simulink model "AGTF30SysDyn_PExPIn"  (R2023b)
settings: Solver=ode4  StartTime=0.0  StopTime=MWS.In.tend  FixedStep=MWS.In.Ts  RelTol=1e-3  EnableMultiTasking=on
model workspace: external: MAT-File (data not in the file)
values from neighbouring files (symbols this model uses):
  MWS = setup_initialize(MWS,startPt,SSsolverSP)    [Setup_Simulation.m]    (also in run_AGTF30e_script.m = Setup_Simulation(inputMethod,MWS.In,filename,Mdl,SSsolverSP))
undefined symbols (not defined in the file or in its folder): DiscIntNeverNeededParam
libraries: simulink x32, Lib_Solve_ModelSource_TMATS x28, Lib_EMTAT x27, Lib_Cntrl_FirstOrderSensor_TMATS x19, Lib_Cntrl_FirstOrderActuator_TMATS x2, Lib_Cntrl_LimitSelect_TMATS x2, Lib_Solve_OuterLoopIntegrator_TMATS x2, Lib_Cntrl_CorrectedSpeed_TMATS x1, Lib_Solve_IterNRSolverJC_TMATS x1, slpidlib x1
(part 7 of 8)

== system AGTF30SysDyn_PExPIn/Control System/Electric Machine Controllers/EM Controllers/PGB EM Control/VEATE EM Controllers/Base Power/Base Power - Boost and PEx/Boost PEx - HC LR CS ==
  note: COUPLING EM
  note: HP - CARRIER , LP - RING, COUPLING - SUN
  note: LP EM
  note: HP EM
  note: MAKE SURE THE POWER DEMAND/LOAD IS BEING
      | PROVIDED. WITH VEATE, CROSS-COUPLING EFFECTS
      | IN THE COMPONENTS CAN RELECT POWER BACK TO
      | OTHER COMPONENTS AND A SMALL DIFFERENCE (A FEW
      | 10'S OF HORSEPOWER) COULDBE OBSERVED. THIS WILL
      | WIPE OUT THE DIFFENCE.
  PwrL_Base : Inport
  PwrH_Base : Inport  Port=2
  K_PXeffL : Inport  Port=3
  K_PXeffH : Inport  Port=4
  NS : Inport  Port=5
  NR : Inport  Port=6
  NC : Inport  Port=7
  Abs : Abs  SaturateOnIntegerOverflow=off
  Abs1 : Abs  SaturateOnIntegerOverflow=off
  Abs2 : Abs  SaturateOnIntegerOverflow=off
  Divide : Product  Inputs=*/
  Divide{2..3,5..7,9..11} (8 alike) : Product  Inputs=**
  Gain1 : Gain  Gain=1/5252.113
  Gain15 : Gain  Gain=1/MWS.Shaft.PGB.Ring.GR_gb %GR_gb = Ngb/Nem
  Gain2 : Gain  Gain=1/5252.113
  Gain3 : Gain  Gain=1/MWS.Shaft.PGB.Carrier.GR_gb %GR_gb = Ngb/Nem
  Gain4 : Gain  Gain=1/5252.113
  Gain5 : Gain  Gain=1/MWS.Shaft.PGB.Sun.GR_gb %GR_gb = Ngb/Nem
  MinMax : MinMax
  MinMax1 : MinMax
  MinMax2 : MinMax
  Mux1 : Mux  Inputs=3
  Mux2 : Mux  Inputs=3
  Mux3 : Mux  Inputs=3
  PwrMax_Base : Constant  Value=MWS.Cntrl.EMR.PwrMax_Base
  PwrMax_Base1 : Constant  Value=MWS.Cntrl.EMC.PwrMax_Base
  PwrMax_Base2 : Constant  Value=MWS.Cntrl.EMS.PwrMax_Base
  Sign : Signum
  Sign1 : Signum
  Sign2 : Signum
  Sum : Sum  Inputs=|+-
  Sum1 : Sum  Inputs=|-+
  Sum5 : Sum  Inputs=|+++
  Sum6 : Sum  Inputs=|++
  Sum7 : Sum  Inputs=|+-
  Sum8 : Sum  Inputs=++|
  TrqMax_Base : Constant  Value=MWS.Cntrl.EMR.TrqMax_Base
  TrqMax_Base1 : Constant  Value=MWS.Cntrl.EMC.TrqMax_Base
  TrqMax_Base2 : Constant  Value=MWS.Cntrl.EMS.TrqMax_Base
  Zero : Constant  Value=0
  PemS_Base : Outport
  PemR_Base : Outport  Port=2
  PemC_Base : Outport  Port=3
  PemP_Base : Outport  Port=4
  wires:
  [KPXeffH] -> Divide9/2
  NS/1 -> Gain5/1
  [KPXeffL] -> Divide5/2
  K_PXeffH/1 -> [KPXeffH]
  K_PXeffL/1 -> [KPXeffL]
  Sum7/1 -> Sum8/1
  [PwrH_Base] -> Sum6/2
  [PwrL_Base] -> Sum6/1
  Sum8/1 -> Mux2/1, Sign2/1
  Sum5/1 -> Sum7/2
  Sum6/1 -> Sum7/1
  PwrL_Base/1 -> Divide/1, [PwrL_Base]
  Divide9/1 -> Sum1/1
  [PemL_Base] -> Sum5/1
  Mux2/1 -> Abs2/1
  TrqMax_Base/1 -> Divide3/1
  Divide3/1 -> Gain1/1
  Sign1/1 -> Divide7/1
  [KPXeffL] -> Divide/2
  [PemCoup_Base] -> Divide5/1
  Sum/1 -> Mux1/1, Sign1/1  "Power to LP from LP EM"
  MinMax1/1 -> Divide7/2
  Abs/1 -> MinMax/1
  PwrMax_Base1/1 -> Mux2/2
  Gain5/1 -> Divide10/2
  PwrMax_Base2/1 -> Mux3/2
  Divide7/1 -> PemR_Base/1, [PemL_Base]
  Mux3/1 -> Abs/1
  Divide/1 -> Mux3/1, Sign/1  "Power to LP from Coupling"
  MinMax/1 -> Divide2/2
  TrqMax_Base2/1 -> Divide10/1
  Divide10/1 -> Gain4/1
  [PwrL_Base] -> Sum/1
  Divide2/1 -> PemS_Base/1, [PemCoup_Base]
  NR/1 -> Gain15/1
  [PemCoup_Base] -> Divide9/1, Sum5/2
  Gain4/1 -> Mux3/3
  Gain3/1 -> Divide6/2
  Gain1/1 -> Mux1/3
  Sum1/1 -> Sum5/3, Sum8/2
  Divide5/1 -> Sum/2
  Gain15/1 -> Divide3/2
  NC/1 -> Gain3/1
  Abs2/1 -> MinMax2/1
  PwrMax_Base/1 -> Mux1/2
  Mux1/1 -> Abs1/1
  Gain2/1 -> Mux2/3
  Divide11/1 -> PemC_Base/1
  Divide6/1 -> Gain2/1
  TrqMax_Base1/1 -> Divide6/1
  MinMax2/1 -> Divide11/2
  Abs1/1 -> MinMax1/1
  Sign/1 -> Divide2/1
  Sign2/1 -> Divide11/1
  PwrH_Base/1 -> Sum1/2, [PwrH_Base]
  Zero/1 -> PemP_Base/1

== system AGTF30SysDyn_PExPIn/Control System/Electric Machine Controllers/EM Controllers/PGB EM Control/VEATE EM Controllers/Base Power/Base Power - Boost and PEx/Boost PEx - HC LS CR ==
  note: MAKE SURE THE POWER DEMAND/LOAD IS BEING
      | PROVIDED. WITH VEATE, CROSS-COUPLING EFFECTS
      | IN THE COMPONENTS CAN RELECT POWER BACK TO
      | OTHER COMPONENTS AND A SMALL DIFFERENCE (A FEW
      | 10'S OF HORSEPOWER) COULDBE OBSERVED. THIS WILL
      | WIPE OUT THE DIFFENCE.
  note: HP EM
  note: LP EM
  note: HP - CARRIER , LP - SUN, COUPLING - RING
  note: COUPLING EM
  PwrL_Base : Inport
  PwrH_Base : Inport  Port=2
  K_PXeffL : Inport  Port=3
  K_PXeffH : Inport  Port=4
  NS : Inport  Port=5
  NR : Inport  Port=6
  NC : Inport  Port=7
  Abs : Abs  SaturateOnIntegerOverflow=off
  Abs1 : Abs  SaturateOnIntegerOverflow=off
  Abs2 : Abs  SaturateOnIntegerOverflow=off
  Divide : Product  Inputs=*/
  Divide{2..3,5..7,9..11} (8 alike) : Product  Inputs=**
  Gain1 : Gain  Gain=1/5252.113
  Gain15 : Gain  Gain=1/MWS.Shaft.PGB.Ring.GR_gb %GR_gb = Ngb/Nem
  Gain2 : Gain  Gain=1/5252.113
  Gain3 : Gain  Gain=1/MWS.Shaft.PGB.Carrier.GR_gb %GR_gb = Ngb/Nem
  Gain4 : Gain  Gain=1/5252.113
  Gain5 : Gain  Gain=1/MWS.Shaft.PGB.Sun.GR_gb %GR_gb = Ngb/Nem
  MinMax : MinMax
  MinMax1 : MinMax
  MinMax2 : MinMax
  Mux1 : Mux  Inputs=3
  Mux2 : Mux  Inputs=3
  Mux3 : Mux  Inputs=3
  PwrMax_Base : Constant  Value=MWS.Cntrl.EMR.PwrMax_Base
  PwrMax_Base1 : Constant  Value=MWS.Cntrl.EMC.PwrMax_Base
  PwrMax_Base2 : Constant  Value=MWS.Cntrl.EMS.PwrMax_Base
  Sign : Signum
  Sign1 : Signum
  Sign2 : Signum
  Sum : Sum  Inputs=|+-
  Sum1 : Sum  Inputs=|-+
  Sum5 : Sum  Inputs=|+++
  Sum6 : Sum  Inputs=|++
  Sum7 : Sum  Inputs=|+-
  Sum8 : Sum  Inputs=++|
  TrqMax_Base : Constant  Value=MWS.Cntrl.EMR.TrqMax_Base
  TrqMax_Base1 : Constant  Value=MWS.Cntrl.EMC.TrqMax_Base
  TrqMax_Base2 : Constant  Value=MWS.Cntrl.EMS.TrqMax_Base
  Zero : Constant  Value=0
  PemS_Base : Outport
  PemR_Base : Outport  Port=2
  PemC_Base : Outport  Port=3
  PemP_Base : Outport  Port=4
  wires:
  Zero/1 -> PemP_Base/1
  PwrH_Base/1 -> [PwrH_Base], Sum1/2
  Sign2/1 -> Divide11/1
  Sign/1 -> Divide2/1
  Abs1/1 -> MinMax1/1
  MinMax2/1 -> Divide11/2
  TrqMax_Base1/1 -> Divide6/1
  Divide6/1 -> Gain2/1
  Divide11/1 -> PemC_Base/1
  Gain2/1 -> Mux2/3
  Mux1/1 -> Abs/1
  PwrMax_Base/1 -> Mux1/2
  Abs2/1 -> MinMax2/1
  NC/1 -> Gain3/1
  Gain15/1 -> Divide3/2
  Divide5/1 -> Sum/2
  Sum1/1 -> Sum8/2, Sum5/3
  Gain1/1 -> Mux1/3
  Gain3/1 -> Divide6/2
  Gain4/1 -> Mux3/3
  [PemCoup_Base] -> Sum5/2, Divide9/1
  NR/1 -> Gain15/1
  Divide2/1 -> PemR_Base/1, [PemCoup_Base]
  [PwrL_Base] -> Sum/1
  Divide10/1 -> Gain4/1
  TrqMax_Base2/1 -> Divide10/1
  MinMax/1 -> Divide2/2
  Divide/1 -> Mux1/1, Sign/1  "Power to LP from Coupling"
  Mux3/1 -> Abs1/1
  Divide7/1 -> PemS_Base/1, [PemL_Base]
  PwrMax_Base2/1 -> Mux3/2
  Gain5/1 -> Divide10/2
  PwrMax_Base1/1 -> Mux2/2
  Abs/1 -> MinMax/1
  MinMax1/1 -> Divide7/2
  Sum/1 -> Sign1/1, Mux3/1  "Power to LP from LP EM"
  [PemCoup_Base] -> Divide5/1
  [KPXeffL] -> Divide/2
  Sign1/1 -> Divide7/1
  Divide3/1 -> Gain1/1
  TrqMax_Base/1 -> Divide3/1
  Mux2/1 -> Abs2/1
  [PemL_Base] -> Sum5/1
  Divide9/1 -> Sum1/1
  PwrL_Base/1 -> [PwrL_Base], Divide/1
  Sum6/1 -> Sum7/1
  Sum5/1 -> Sum7/2
  Sum8/1 -> Mux2/1, Sign2/1
  [PwrL_Base] -> Sum6/1
  [PwrH_Base] -> Sum6/2
  Sum7/1 -> Sum8/1
  K_PXeffL/1 -> [KPXeffL]
  K_PXeffH/1 -> [KPXeffH]
  [KPXeffL] -> Divide5/2
  NS/1 -> Gain5/1
  [KPXeffH] -> Divide9/2

== system AGTF30SysDyn_PExPIn/Control System/Electric Machine Controllers/EM Controllers/PGB EM Control/VEATE EM Controllers/Base Power/Base Power - Boost and PEx/Boost PEx - HR LC CS ==
  note: COUPLING EM
  note: HP - RING, LP - CARRIER, COUPLING - SUN
  note: LP EM
  note: HP EM
  note: MAKE SURE THE POWER DEMAND/LOAD IS BEING
      | PROVIDED. WITH VEATE, CROSS-COUPLING EFFECTS
      | IN THE COMPONENTS CAN RELECT POWER BACK TO
      | OTHER COMPONENTS AND A SMALL DIFFERENCE (A FEW
      | 10'S OF HORSEPOWER) COULDBE OBSERVED. THIS WILL
      | WIPE OUT THE DIFFENCE.
  PwrL_Base : Inport
  PwrH_Base : Inport  Port=2
  K_PXeffL : Inport  Port=3
  K_PXeffH : Inport  Port=4
  NS : Inport  Port=5
  NR : Inport  Port=6
  NC : Inport  Port=7
  Abs : Abs  SaturateOnIntegerOverflow=off
  Abs1 : Abs  SaturateOnIntegerOverflow=off
  Abs2 : Abs  SaturateOnIntegerOverflow=off
  Compare To Constant : simulink/Logic and Bit Operations/Compare To Constant  relop===  const=3.0  OutDataTypeStr=boolean
  Const : Constant  Value=0
  Const1 : Constant  Value=MWS.In.Options.HybridConfig
  Divide : Product  Inputs=*/
  Divide{2..3,5..7,9..11} (8 alike) : Product  Inputs=**
  Gain1 : Gain  Gain=1/5252.113
  Gain15 : Gain  Gain=1/MWS.Shaft.PGB.Ring.GR_gb %GR_gb = Ngb/Nem
  Gain2 : Gain  Gain=1/5252.113
  Gain3 : Gain  Gain=1/MWS.Shaft.PGB.Carrier.GR_gb %GR_gb = Ngb/Nem
  Gain4 : Gain  Gain=1/5252.113
  Gain5 : Gain  Gain=1/MWS.Shaft.PGB.Sun.GR_gb %GR_gb = Ngb/Nem
  MinMax : MinMax
  MinMax1 : MinMax
  MinMax2 : MinMax
  Mux1 : Mux  Inputs=3
  Mux2 : Mux  Inputs=3
  Mux3 : Mux  Inputs=3
  PwrMax_Base : Constant  Value=MWS.Cntrl.EMR.PwrMax_Base
  PwrMax_Base1 : Constant  Value=MWS.Cntrl.EMC.PwrMax_Base
  PwrMax_Base2 : Constant  Value=MWS.Cntrl.EMS.PwrMax_Base
  Sign : Signum
  Sign1 : Signum
  Sign2 : Signum
  Sum : Sum  Inputs=|+-
  Sum1 : Sum  Inputs=|-+
  Sum5 : Sum  Inputs=|+++
  Sum6 : Sum  Inputs=|++
  Sum7 : Sum  Inputs=|+-
  Sum8 : Sum  Inputs=++|
  Switch : Switch  Criteria=u2 > Threshold  SaturateOnIntegerOverflow=off  InputSameDT=off
  TrqMax_Base : Constant  Value=MWS.Cntrl.EMR.TrqMax_Base
  TrqMax_Base1 : Constant  Value=MWS.Cntrl.EMC.TrqMax_Base
  TrqMax_Base2 : Constant  Value=MWS.Cntrl.EMS.TrqMax_Base
  Zero : Constant  Value=0
  PemS_Base : Outport
  PemR_Base : Outport  Port=2
  PemC_Base : Outport  Port=3
  PemP_Base : Outport  Port=4
  wires:
  [KPXeffH] -> Divide9/2
  NS/1 -> Gain5/1
  [KPXeffL] -> Divide5/2
  K_PXeffH/1 -> [KPXeffH]
  K_PXeffL/1 -> [KPXeffL]
  Sum7/1 -> Sum8/1
  [PwrH_Base] -> Sum6/2
  [PwrL_Base] -> Sum6/1
  Sum8/1 -> Mux1/1, Sign2/1
  Sum5/1 -> Sum7/2
  Sum6/1 -> Sum7/1
  PwrL_Base/1 -> Divide/1, [PwrL_Base]
  Divide9/1 -> Sum1/1
  [PemL_Base] -> Sum5/1
  Mux2/1 -> Abs1/1
  TrqMax_Base/1 -> Divide3/1
  Divide3/1 -> Gain1/1
  Sign1/1 -> Divide7/1
  [KPXeffL] -> Divide/2
  [PemCoup_Base] -> Divide5/1
  Sum/1 -> Mux2/1, Sign1/1  "Power to LP from LP EM"
  MinMax1/1 -> Divide7/2
  Abs/1 -> MinMax/1
  PwrMax_Base1/1 -> Mux2/2
  Gain5/1 -> Divide10/2
  Divide7/1 -> PemC_Base/1, [PemL_Base]
  Mux3/1 -> Abs/1
  Divide/1 -> Mux3/1, Sign/1  "Power to LP from Coupling"
  MinMax/1 -> Divide2/2
  TrqMax_Base2/1 -> Divide10/1
  Divide10/1 -> Gain4/1
  [PwrL_Base] -> Sum/1
  Divide2/1 -> PemS_Base/1, [PemCoup_Base]
  NR/1 -> Gain15/1
  [PemCoup_Base] -> Divide9/1, Sum5/2
  Gain4/1 -> Mux3/3
  Gain3/1 -> Divide6/2
  Gain1/1 -> Mux1/3
  Sum1/1 -> Sum5/3, Sum8/2
  Divide5/1 -> Sum/2
  Gain15/1 -> Divide3/2
  NC/1 -> Gain3/1
  Abs2/1 -> MinMax2/1
  PwrMax_Base/1 -> Mux1/2
  Mux1/1 -> Abs2/1
  Gain2/1 -> Mux2/3
  Divide11/1 -> PemR_Base/1
  Divide6/1 -> Gain2/1
  TrqMax_Base1/1 -> Divide6/1
  MinMax2/1 -> Divide11/2
  Abs1/1 -> MinMax1/1
  Sign/1 -> Divide2/1
  Sign2/1 -> Divide11/1
  PwrH_Base/1 -> Sum1/2, [PwrH_Base]
  Zero/1 -> PemP_Base/1
  Const1/1 -> Compare To Constant/1
  Compare To Constant/1 -> Switch/2
  Switch/1 -> Mux3/2
  PwrMax_Base2/1 -> Switch/3
  Const/1 -> Switch/1

== system AGTF30SysDyn_PExPIn/Control System/Electric Machine Controllers/EM Controllers/PGB EM Control/VEATE EM Controllers/Base Power/Base Power - Boost and PEx/Boost PEx - HR LS CC ==
  note: MAKE SURE THE POWER DEMAND/LOAD IS BEING
      | PROVIDED. WITH VEATE, CROSS-COUPLING EFFECTS
      | IN THE COMPONENTS CAN RELECT POWER BACK TO
      | OTHER COMPONENTS AND A SMALL DIFFERENCE (A FEW
      | 10'S OF HORSEPOWER) COULDBE OBSERVED. THIS WILL
      | WIPE OUT THE DIFFENCE.
  note: HP EM
  note: LP EM
  note: HP - RING, LP - SUN, COUPLING - CARRIER
  note: COUPLING EM
  PwrL_Base : Inport
  PwrH_Base : Inport  Port=2
  K_PXeffL : Inport  Port=3
  K_PXeffH : Inport  Port=4
  NS : Inport  Port=5
  NR : Inport  Port=6
  NC : Inport  Port=7
  Abs : Abs  SaturateOnIntegerOverflow=off
  Abs1 : Abs  SaturateOnIntegerOverflow=off
  Abs2 : Abs  SaturateOnIntegerOverflow=off
  Divide : Product  Inputs=*/
  Divide{2..3,5..7,9..11} (8 alike) : Product  Inputs=**
  Gain1 : Gain  Gain=1/5252.113
  Gain15 : Gain  Gain=1/MWS.Shaft.PGB.Ring.GR_gb %GR_gb = Ngb/Nem
  Gain2 : Gain  Gain=1/5252.113
  Gain3 : Gain  Gain=1/MWS.Shaft.PGB.Carrier.GR_gb %GR_gb = Ngb/Nem
  Gain4 : Gain  Gain=1/5252.113
  Gain5 : Gain  Gain=1/MWS.Shaft.PGB.Sun.GR_gb %GR_gb = Ngb/Nem
  MinMax : MinMax
  MinMax1 : MinMax
  MinMax2 : MinMax
  Mux1 : Mux  Inputs=3
  Mux2 : Mux  Inputs=3
  Mux3 : Mux  Inputs=3
  PwrMax_Base : Constant  Value=MWS.Cntrl.EMR.PwrMax_Base
  PwrMax_Base1 : Constant  Value=MWS.Cntrl.EMC.PwrMax_Base
  PwrMax_Base2 : Constant  Value=MWS.Cntrl.EMS.PwrMax_Base
  Sign : Signum
  Sign1 : Signum
  Sign2 : Signum
  Sum : Sum  Inputs=|+-
  Sum1 : Sum  Inputs=|-+
  Sum5 : Sum  Inputs=|+++
  Sum6 : Sum  Inputs=|++
  Sum7 : Sum  Inputs=|+-
  Sum8 : Sum  Inputs=++|
  TrqMax_Base : Constant  Value=MWS.Cntrl.EMR.TrqMax_Base
  TrqMax_Base1 : Constant  Value=MWS.Cntrl.EMC.TrqMax_Base
  TrqMax_Base2 : Constant  Value=MWS.Cntrl.EMS.TrqMax_Base
  Zero : Constant  Value=0
  PemS_Base : Outport
  PemR_Base : Outport  Port=2
  PemC_Base : Outport  Port=3
  PemP_Base : Outport  Port=4
  wires:
  Zero/1 -> PemP_Base/1
  PwrH_Base/1 -> [PwrH_Base], Sum1/2
  Sign2/1 -> Divide11/1
  Sign/1 -> Divide2/1
  Abs1/1 -> MinMax1/1
  MinMax2/1 -> Divide11/2
  TrqMax_Base1/1 -> Divide6/1
  Divide6/1 -> Gain2/1
  Divide11/1 -> PemR_Base/1
  Gain2/1 -> Mux2/3
  Mux1/1 -> Abs2/1
  PwrMax_Base/1 -> Mux1/2
  Abs2/1 -> MinMax2/1
  NC/1 -> Gain3/1
  Gain15/1 -> Divide3/2
  Divide5/1 -> Sum/2
  Sum1/1 -> Sum8/2, Sum5/3
  Gain1/1 -> Mux1/3
  Gain3/1 -> Divide6/2
  Gain4/1 -> Mux3/3
  [PemCoup_Base] -> Sum5/2, Divide9/1
  NR/1 -> Gain15/1
  Divide2/1 -> PemC_Base/1, [PemCoup_Base]
  [PwrL_Base] -> Sum/1
  Divide10/1 -> Gain4/1
  TrqMax_Base2/1 -> Divide10/1
  MinMax/1 -> Divide2/2
  Divide/1 -> Sign/1, Mux2/1  "Power to LP from Coupling"
  Mux3/1 -> Abs1/1
  Divide7/1 -> PemS_Base/1, [PemL_Base]
  PwrMax_Base2/1 -> Mux3/2
  Gain5/1 -> Divide10/2
  PwrMax_Base1/1 -> Mux2/2
  Abs/1 -> MinMax/1
  MinMax1/1 -> Divide7/2
  Sum/1 -> Mux3/1, Sign1/1  "Power to LP from LP EM"
  [PemCoup_Base] -> Divide5/1
  [KPXeffL] -> Divide/2
  Sign1/1 -> Divide7/1
  Divide3/1 -> Gain1/1
  TrqMax_Base/1 -> Divide3/1
  Mux2/1 -> Abs/1
  [PemL_Base] -> Sum5/1
  Divide9/1 -> Sum1/1
  PwrL_Base/1 -> [PwrL_Base], Divide/1
  Sum6/1 -> Sum7/1
  Sum5/1 -> Sum7/2
  Sum8/1 -> Mux1/1, Sign2/1
  [PwrL_Base] -> Sum6/1
  [PwrH_Base] -> Sum6/2
  Sum7/1 -> Sum8/1
  K_PXeffL/1 -> [KPXeffL]
  K_PXeffH/1 -> [KPXeffH]
  [KPXeffL] -> Divide5/2
  NS/1 -> Gain5/1
  [KPXeffH] -> Divide9/2

== system AGTF30SysDyn_PExPIn/Control System/Electric Machine Controllers/EM Controllers/PGB EM Control/VEATE EM Controllers/Base Power/Base Power - Boost and PEx/Boost PEx - HS LC CR ==
  note: MAKE SURE THE POWER DEMAND/LOAD IS BEING
      | PROVIDED. WITH VEATE, CROSS-COUPLING EFFECTS
      | IN THE COMPONENTS CAN RELECT POWER BACK TO
      | OTHER COMPONENTS AND A SMALL DIFFERENCE (A FEW
      | 10'S OF HORSEPOWER) COULDBE OBSERVED. THIS WILL
      | WIPE OUT THE DIFFENCE.
  note: HP EM
  note: LP EM
  note: HP - SUN, LP - CARRIER, COUPLING - RING
  note: COUPLING EM
  PwrL_Base : Inport
  PwrH_Base : Inport  Port=2
  K_PXeffL : Inport  Port=3
  K_PXeffH : Inport  Port=4
  NS : Inport  Port=5
  NR : Inport  Port=6
  NC : Inport  Port=7
  Abs : Abs  SaturateOnIntegerOverflow=off
  Abs1 : Abs  SaturateOnIntegerOverflow=off
  Abs2 : Abs  SaturateOnIntegerOverflow=off
  Compare To Constant : simulink/Logic and Bit Operations/Compare To Constant  relop===  const=3.0  OutDataTypeStr=boolean
  Const : Constant  Value=0
  Const1 : Constant  Value=MWS.In.Options.HybridConfig
  Divide : Product  Inputs=*/
  Divide{2..3,5..7,9..11} (8 alike) : Product  Inputs=**
  Gain1 : Gain  Gain=1/5252.113
  Gain15 : Gain  Gain=1/MWS.Shaft.PGB.Ring.GR_gb %GR_gb = Ngb/Nem
  Gain2 : Gain  Gain=1/5252.113
  Gain3 : Gain  Gain=1/MWS.Shaft.PGB.Carrier.GR_gb %GR_gb = Ngb/Nem
  Gain4 : Gain  Gain=1/5252.113
  Gain5 : Gain  Gain=1/MWS.Shaft.PGB.Sun.GR_gb %GR_gb = Ngb/Nem
  MinMax : MinMax
  MinMax1 : MinMax
  MinMax2 : MinMax
  Mux1 : Mux  Inputs=3
  Mux2 : Mux  Inputs=3
  Mux3 : Mux  Inputs=3
  PwrMax_Base : Constant  Value=MWS.Cntrl.EMR.PwrMax_Base
  PwrMax_Base1 : Constant  Value=MWS.Cntrl.EMC.PwrMax_Base
  PwrMax_Base2 : Constant  Value=MWS.Cntrl.EMS.PwrMax_Base
  Sign : Signum
  Sign1 : Signum
  Sign2 : Signum
  Sum : Sum  Inputs=|+-
  Sum1 : Sum  Inputs=|-+
  Sum5 : Sum  Inputs=|+++
  Sum6 : Sum  Inputs=|++
  Sum7 : Sum  Inputs=|+-
  Sum8 : Sum  Inputs=++|
  Switch : Switch  Criteria=u2 > Threshold  SaturateOnIntegerOverflow=off  InputSameDT=off
  TrqMax_Base : Constant  Value=MWS.Cntrl.EMR.TrqMax_Base
  TrqMax_Base1 : Constant  Value=MWS.Cntrl.EMC.TrqMax_Base
  TrqMax_Base2 : Constant  Value=MWS.Cntrl.EMS.TrqMax_Base
  Zero : Constant  Value=0
  PemS_Base : Outport
  PemR_Base : Outport  Port=2
  PemC_Base : Outport  Port=3
  PemP_Base : Outport  Port=4
  wires:
  Zero/1 -> PemP_Base/1
  PwrH_Base/1 -> [PwrH_Base], Sum1/2
  Sign2/1 -> Divide11/1
  Sign/1 -> Divide2/1
  Abs1/1 -> MinMax1/1
  MinMax2/1 -> Divide11/2
  TrqMax_Base1/1 -> Divide6/1
  Divide6/1 -> Gain2/1
  Divide11/1 -> PemS_Base/1
  Gain2/1 -> Mux2/3
  Mux1/1 -> Abs/1
  Abs2/1 -> MinMax2/1
  NC/1 -> Gain3/1
  Gain15/1 -> Divide3/2
  Divide5/1 -> Sum/2
  Sum1/1 -> Sum8/2, Sum5/3
  Gain1/1 -> Mux1/3
  Gain3/1 -> Divide6/2
  Gain4/1 -> Mux3/3
  [PemCoup_Base] -> Sum5/2, Divide9/1
  NR/1 -> Gain15/1
  Divide2/1 -> [PemCoup_Base], PemR_Base/1
  [PwrL_Base] -> Sum/1
  Divide10/1 -> Gain4/1
  TrqMax_Base2/1 -> Divide10/1
  MinMax/1 -> Divide2/2
  Divide/1 -> Sign/1, Mux1/1  "Power to LP from Coupling"
  Mux3/1 -> Abs2/1
  Divide7/1 -> [PemL_Base], PemC_Base/1
  PwrMax_Base2/1 -> Mux3/2
  Gain5/1 -> Divide10/2
  PwrMax_Base1/1 -> Mux2/2
  Abs/1 -> MinMax/1
  MinMax1/1 -> Divide7/2
  Sum/1 -> Sign1/1, Mux2/1  "Power to LP from LP EM"
  [PemCoup_Base] -> Divide5/1
  [KPXeffL] -> Divide/2
  Sign1/1 -> Divide7/1
  Divide3/1 -> Gain1/1
  TrqMax_Base/1 -> Divide3/1
  Mux2/1 -> Abs1/1
  [PemL_Base] -> Sum5/1
  Divide9/1 -> Sum1/1
  PwrL_Base/1 -> [PwrL_Base], Divide/1
  Sum6/1 -> Sum7/1
  Sum5/1 -> Sum7/2
  Sum8/1 -> Mux3/1, Sign2/1
  [PwrL_Base] -> Sum6/1
  [PwrH_Base] -> Sum6/2
  Sum7/1 -> Sum8/1
  K_PXeffL/1 -> [KPXeffL]
  K_PXeffH/1 -> [KPXeffH]
  [KPXeffL] -> Divide5/2
  NS/1 -> Gain5/1
  [KPXeffH] -> Divide9/2
  Const/1 -> Switch/1
  Switch/1 -> Mux1/2
  Compare To Constant/1 -> Switch/2
  PwrMax_Base/1 -> Switch/3
  Const1/1 -> Compare To Constant/1

== system AGTF30SysDyn_PExPIn/Control System/Electric Machine Controllers/EM Controllers/PGB EM Control/VEATE EM Controllers/Base Power/Base Power - Boost and PEx/Boost PEx - HS LR CC ==
  note: MAKE SURE THE POWER DEMAND/LOAD IS BEING
      | PROVIDED. WITH VEATE, CROSS-COUPLING EFFECTS
      | IN THE COMPONENTS CAN RELECT POWER BACK TO
      | OTHER COMPONENTS AND A SMALL DIFFERENCE (A FEW
      | 10'S OF HORSEPOWER) COULDBE OBSERVED. THIS WILL
      | WIPE OUT THE DIFFENCE.
  note: HP EM
  note: LP EM
  note: HP - SUN, LP - RING, COUPLING - CARRIER
  note: COUPLING EM
  PwrL_Base : Inport
  PwrH_Base : Inport  Port=2
  K_PXeffL : Inport  Port=3
  K_PXeffH : Inport  Port=4
  NS : Inport  Port=5
  NR : Inport  Port=6
  NC : Inport  Port=7
  Abs : Abs  SaturateOnIntegerOverflow=off
  Abs1 : Abs  SaturateOnIntegerOverflow=off
  Abs2 : Abs  SaturateOnIntegerOverflow=off
  Compare To Constant : simulink/Logic and Bit Operations/Compare To Constant  relop===  const=3.0  OutDataTypeStr=boolean
  Const : Constant  Value=0
  Const1 : Constant  Value=MWS.In.Options.HybridConfig
  Divide : Product  Inputs=*/
  Divide{2..3,5..7,9..11} (8 alike) : Product  Inputs=**
  Gain1 : Gain  Gain=1/5252.113
  Gain15 : Gain  Gain=1/MWS.Shaft.PGB.Ring.GR_gb %GR_gb = Ngb/Nem
  Gain2 : Gain  Gain=1/5252.113
  Gain3 : Gain  Gain=1/MWS.Shaft.PGB.Carrier.GR_gb %GR_gb = Ngb/Nem
  Gain4 : Gain  Gain=1/5252.113
  Gain5 : Gain  Gain=1/MWS.Shaft.PGB.Sun.GR_gb %GR_gb = Ngb/Nem
  MinMax : MinMax
  MinMax1 : MinMax
  MinMax2 : MinMax
  Mux1 : Mux  Inputs=3
  Mux2 : Mux  Inputs=3
  Mux3 : Mux  Inputs=3
  PwrMax_Base : Constant  Value=MWS.Cntrl.EMR.PwrMax_Base
  PwrMax_Base1 : Constant  Value=MWS.Cntrl.EMC.PwrMax_Base
  PwrMax_Base2 : Constant  Value=MWS.Cntrl.EMS.PwrMax_Base
  Sign : Signum
  Sign1 : Signum
  Sign2 : Signum
  Sum : Sum  Inputs=|+-
  Sum1 : Sum  Inputs=|-+
  Sum5 : Sum  Inputs=|+++
  Sum6 : Sum  Inputs=|++
  Sum7 : Sum  Inputs=|+-
  Sum8 : Sum  Inputs=++|
  Switch : Switch  Criteria=u2 > Threshold  SaturateOnIntegerOverflow=off  InputSameDT=off
  TrqMax_Base : Constant  Value=MWS.Cntrl.EMR.TrqMax_Base
  TrqMax_Base1 : Constant  Value=MWS.Cntrl.EMC.TrqMax_Base
  TrqMax_Base2 : Constant  Value=MWS.Cntrl.EMS.TrqMax_Base
  Zero : Constant  Value=0
  PemS_Base : Outport
  PemR_Base : Outport  Port=2
  PemC_Base : Outport  Port=3
  PemP_Base : Outport  Port=4
  wires:
  Zero/1 -> PemP_Base/1
  PwrH_Base/1 -> [PwrH_Base], Sum1/2
  Sign2/1 -> Divide11/1
  Sign/1 -> Divide2/1
  Abs1/1 -> MinMax1/1
  MinMax2/1 -> Divide11/2
  TrqMax_Base1/1 -> Divide6/1
  Divide6/1 -> Gain2/1
  Divide11/1 -> PemS_Base/1
  Gain2/1 -> Mux2/3
  Mux1/1 -> Abs1/1
  PwrMax_Base/1 -> Mux1/2
  Abs2/1 -> MinMax2/1
  NC/1 -> Gain3/1
  Gain15/1 -> Divide3/2
  Divide5/1 -> Sum/2
  Sum1/1 -> Sum8/2, Sum5/3
  Gain1/1 -> Mux1/3
  Gain3/1 -> Divide6/2
  Gain4/1 -> Mux3/3
  [PemCoup_Base] -> Sum5/2, Divide9/1
  NR/1 -> Gain15/1
  Divide2/1 -> PemC_Base/1, [PemCoup_Base]
  [PwrL_Base] -> Sum/1
  Divide10/1 -> Gain4/1
  TrqMax_Base2/1 -> Divide10/1
  MinMax/1 -> Divide2/2
  Divide/1 -> Mux2/1, Sign/1  "Power to LP from Coupling"
  Mux3/1 -> Abs2/1
  Divide7/1 -> PemR_Base/1, [PemL_Base]
  PwrMax_Base2/1 -> Mux3/2
  Gain5/1 -> Divide10/2
  PwrMax_Base1/1 -> Switch/3
  Abs/1 -> MinMax/1
  MinMax1/1 -> Divide7/2
  Sum/1 -> Mux1/1, Sign1/1  "Power to LP from LP EM"
  [PemCoup_Base] -> Divide5/1
  [KPXeffL] -> Divide/2
  Sign1/1 -> Divide7/1
  Divide3/1 -> Gain1/1
  TrqMax_Base/1 -> Divide3/1
  Mux2/1 -> Abs/1
  [PemL_Base] -> Sum5/1
  Divide9/1 -> Sum1/1
  PwrL_Base/1 -> [PwrL_Base], Divide/1
  Sum6/1 -> Sum7/1
  Sum5/1 -> Sum7/2
  Sum8/1 -> Mux3/1, Sign2/1
  [PwrL_Base] -> Sum6/1
  [PwrH_Base] -> Sum6/2
  Sum7/1 -> Sum8/1
  K_PXeffL/1 -> [KPXeffL]
  K_PXeffH/1 -> [KPXeffH]
  [KPXeffL] -> Divide5/2
  NS/1 -> Gain5/1
  [KPXeffH] -> Divide9/2
  Const1/1 -> Compare To Constant/1
  Compare To Constant/1 -> Switch/2
  Const/1 -> Switch/1
  Switch/1 -> Mux2/2

== system AGTF30SysDyn_PExPIn/Control System/Electric Machine Controllers/EM Controllers/PGB EM Control/VEATE EM Controllers/Base Power/Base Power - Standard/Standard - HC ==
  note: HP EM
  note: LP EM / COUPLING EM
  note: HP - CARRIER
  note: COUPLING EM / LP EM
  PwrH_Base : Inport
  NS : Inport  Port=2
  Abs2 : Abs  SaturateOnIntegerOverflow=off
  Divide10 : Product  Inputs=**
  Divide11 : Product  Inputs=**
  Gain4 : Gain  Gain=1/5252.113
  Gain5 : Gain  Gain=1/MWS.Shaft.PGB.Carrier.GR_gb %GR_gb = Ngb/Nem
  MinMax2 : MinMax
  Mux3 : Mux  Inputs=3
  PwrMax_Base2 : Constant  Value=MWS.Cntrl.EMC.PwrMax_Base
  Sign2 : Signum
  TrqMax_Base2 : Constant  Value=MWS.Cntrl.EMC.TrqMax_Base
  Zero : Constant  Value=0
  Zero1 : Constant  Value=0
  Zero2 : Constant  Value=0
  PemS_Base : Outport
  PemR_Base : Outport  Port=2
  PemC_Base : Outport  Port=3
  PemP_Base : Outport  Port=4
  wires:
  Zero/1 -> PemP_Base/1
  Sign2/1 -> Divide11/1
  MinMax2/1 -> Divide11/2
  Divide11/1 -> PemC_Base/1
  Abs2/1 -> MinMax2/1
  PwrH_Base/1 -> Mux3/1, Sign2/1
  Gain4/1 -> Mux3/3
  Zero1/1 -> PemR_Base/1
  Divide10/1 -> Gain4/1
  TrqMax_Base2/1 -> Divide10/1
  Mux3/1 -> Abs2/1
  NS/1 -> Gain5/1
  Zero2/1 -> PemS_Base/1
  PwrMax_Base2/1 -> Mux3/2
  Gain5/1 -> Divide10/2

== system AGTF30SysDyn_PExPIn/Control System/Electric Machine Controllers/EM Controllers/PGB EM Control/VEATE EM Controllers/Base Power/Base Power - Standard/Standard - HR ==
  note: COUPLING EM / LP EM
  note: HP - RING
  note: LP EM / COUPLING EM
  note: HP EM
  PwrH_Base : Inport
  NR : Inport  Port=2
  Abs2 : Abs  SaturateOnIntegerOverflow=off
  Divide10 : Product  Inputs=**
  Divide11 : Product  Inputs=**
  Gain4 : Gain  Gain=1/5252.113
  Gain5 : Gain  Gain=1/MWS.Shaft.PGB.Ring.GR_gb %GR_gb = Ngb/Nem
  MinMax2 : MinMax
  Mux3 : Mux  Inputs=3
  PwrMax_Base2 : Constant  Value=MWS.Cntrl.EMR.PwrMax_Base
  Sign2 : Signum
  TrqMax_Base2 : Constant  Value=MWS.Cntrl.EMR.TrqMax_Base
  Zero : Constant  Value=0
  Zero1 : Constant  Value=0
  Zero2 : Constant  Value=0
  PemS_Base : Outport
  PemR_Base : Outport  Port=2
  PemC_Base : Outport  Port=3
  PemP_Base : Outport  Port=4
  wires:
  Gain5/1 -> Divide10/2
  PwrMax_Base2/1 -> Mux3/2
  Zero2/1 -> PemS_Base/1
  NR/1 -> Gain5/1
  Mux3/1 -> Abs2/1
  TrqMax_Base2/1 -> Divide10/1
  Divide10/1 -> Gain4/1
  Zero1/1 -> PemC_Base/1
  Gain4/1 -> Mux3/3
  PwrH_Base/1 -> Sign2/1, Mux3/1
  Abs2/1 -> MinMax2/1
  Divide11/1 -> PemR_Base/1
  MinMax2/1 -> Divide11/2
  Sign2/1 -> Divide11/1
  Zero/1 -> PemP_Base/1

== system AGTF30SysDyn_PExPIn/Control System/Electric Machine Controllers/EM Controllers/PGB EM Control/VEATE EM Controllers/Base Power/Base Power - Standard/Standard - HS ==
  note: HP EM
  note: LP EM / COUPLING EM
  note: HP - SUN
  note: COUPLING EM / LP EM
  PwrH_Base : Inport
  NS : Inport  Port=2
  Abs2 : Abs  SaturateOnIntegerOverflow=off
  Divide10 : Product  Inputs=**
  Divide11 : Product  Inputs=**
  Gain4 : Gain  Gain=1/5252.113
  Gain5 : Gain  Gain=1/MWS.Shaft.PGB.Sun.GR_gb %GR_gb = Ngb/Nem
  MinMax2 : MinMax
  Mux3 : Mux  Inputs=3
  PwrMax_Base2 : Constant  Value=MWS.Cntrl.EMS.PwrMax_Base
  Sign2 : Signum
  TrqMax_Base2 : Constant  Value=MWS.Cntrl.EMS.TrqMax_Base
  Zero : Constant  Value=0
  Zero1 : Constant  Value=0
  Zero2 : Constant  Value=0
  PemS_Base : Outport
  PemR_Base : Outport  Port=2
  PemC_Base : Outport  Port=3
  PemP_Base : Outport  Port=4
  wires:
  Zero/1 -> PemP_Base/1
  Sign2/1 -> Divide11/1
  MinMax2/1 -> Divide11/2
  Divide11/1 -> PemS_Base/1
  Abs2/1 -> MinMax2/1
  PwrH_Base/1 -> Mux3/1, Sign2/1
  Gain4/1 -> Mux3/3
  Zero1/1 -> PemC_Base/1
  Divide10/1 -> Gain4/1
  TrqMax_Base2/1 -> Divide10/1
  Mux3/1 -> Abs2/1
  NS/1 -> Gain5/1
  Zero2/1 -> PemR_Base/1
  PwrMax_Base2/1 -> Mux3/2
  Gain5/1 -> Divide10/2

== system AGTF30SysDyn_PExPIn/Control System/Electric Machine Controllers/EM Controllers/PGB EM Control/VEATE EM Controllers/TEEM Power/TEEM Power/TEEM - HC LR CS ==
  note: COUPLING EM
  note: HP - CARRIER, LP - RING, COUPLING - SUN
  note: LP EM
  note: HP EM
  PwrInAccel : Inport
  PwrExAccel : Inport  Port=2
  PwrXDecel : Inport  Port=3
  K_PXeffH : Inport  Port=4
  K_PXeffL : Inport  Port=5
  transientType : Inport  Port=6
  Abs : Abs  SaturateOnIntegerOverflow=off
  Abs1 : Abs  SaturateOnIntegerOverflow=off
  Abs2 : Abs  SaturateOnIntegerOverflow=off
  Divide : Product  Inputs=*/
  Divide{2,5,9,11} (4 alike) : Product  Inputs=**
  Divide4 : Product  Inputs=*/
  Divide6 : Product  Inputs=*/
  Gain : Gain  Gain=-1
  Gain2 : Gain  Gain=-1
  Gain3 : Gain  Gain=-1
  MinMax : MinMax
  MinMax2 : MinMax
  Mux1 : Mux  Inputs=2
  Mux3 : Mux  Inputs=2
  PwrMax_TEEM : Constant  Value=MWS.PowerSystem.PwrMaxCoup_TEEMa
  PwrMax_TEEM1 : Constant  Value=MWS.PowerSystem.PwrMaxH_TEEM  VectorParams1D=off
  PwrMax_TEEM2 : Constant  Value=MWS.PowerSystem.PwrMaxCoup_TEEMd
  Rate Limiter : RateLimiter  RisingSlewLimit=inf  FallingSlewLimit=-MWS.PowerSystem.PwrMaxCoup_TEEMa/0.8  SampleTimeMode=inherited
  Relational Operator : RelationalOperator  Operator=>  OutDataTypeStr=boolean  RndMeth=Simplest  InputSameDT=off
  Sign : Signum
  Sign2 : Signum
  Sum1 : Sum  Inputs=|-+
  Sum2 : Sum  Inputs=|-+
  Sum3 : Sum  Inputs=|+-
  Sum4 : Sum  Inputs=|+-
  Switch{,1..4} (5 alike) : Switch  Criteria=u2 > Threshold  SaturateOnIntegerOverflow=off  InputSameDT=off
  Terminator : Terminator
  Terminator1 : Terminator
  Zero : Constant  Value=0
  Zero1 : Constant
  Zero2 : Constant
  zero : Constant  Value=0
  PemS_TEEM : Outport
  PemR_TEEM : Outport  Port=2
  PemC_TEEM : Outport  Port=3
  PemP_TEEM : Outport  Port=4
  wires:
  Abs/1 -> MinMax/1
  PwrMax_TEEM1/1 -> Mux3/2
  zero/1 -> PemR_TEEM/1
  Mux3/1 -> Abs2/1
  Switch/1 -> Sign/1, Mux1/1  "Power of Coupling EM"
  MinMax/1 -> Divide2/2
  Switch1/1 -> Mux3/1, Sign2/1
  Abs2/1 -> MinMax2/1
  Mux1/1 -> Abs/1
  Divide11/1 -> PemC_TEEM/1
  MinMax2/1 -> Divide11/2
  Sign/1 -> Divide2/1
  Sign2/1 -> Divide11/1
  Divide9/1 -> Sum1/1
  [PwrInAccel] -> Sum1/2
  Zero/1 -> PemP_TEEM/1
  Divide2/1 -> Rate Limiter/1, Switch4/3
  PwrInAccel/1 -> [PwrInAccel]
  PwrXDecel/1 -> [PwrXDecel]
  K_PXeffH/1 -> [K_PXeffH]
  [K_PXeffH] -> Divide/2
  [K_PXeffH] -> Divide9/2
  transientType/1 -> [transientType]
  Sum1/1 -> Switch1/1
  [transientType] -> Switch1/2
  Gain/1 -> Switch1/3
  Switch2/1 -> Mux1/2
  PwrMax_TEEM/1 -> Switch2/1
  PwrMax_TEEM2/1 -> Switch2/3
  [transientType] -> Switch/2, Switch2/2
  K_PXeffL/1 -> Terminator1/1
  Divide/1 -> Switch/1
  PwrExAccel/1 -> Terminator/1
  [PemCoup_Base] -> Gain/1, Divide9/1
  [PwrInAccel] -> Divide/1
  [K_PXeffH] -> Divide5/2
  Rate Limiter/1 -> Switch3/3, Divide5/1, Abs1/1  "PCoup"
  [PwrInAccel] -> Sum2/2
  Divide5/1 -> Sum2/1  "PwrXL2H"
  Sum2/1 -> Relational Operator/2  "PH"
  Relational Operator/1 -> Switch3/2
  Switch3/1 -> Switch4/1
  Zero1/1 -> Sum3/1
  [K_PXeffH] -> Sum3/2
  Sum3/1 -> Divide6/2
  [PwrInAccel] -> Divide6/1
  Divide6/1 -> Gain2/1
  Abs1/1 -> Relational Operator/1
  Gain2/1 -> Switch3/1
  Switch4/1 -> PemS_TEEM/1, [PemCoup_Base]  "Power of Coupling EM"
  [transientType] -> Switch4/2
  Gain3/1 -> Switch/3
  Divide4/1 -> Gain3/1
  Zero2/1 -> Sum4/1
  [K_PXeffH] -> Sum4/2
  Sum4/1 -> Divide4/2
  [PwrXDecel] -> Divide4/1

== system AGTF30SysDyn_PExPIn/Control System/Electric Machine Controllers/EM Controllers/PGB EM Control/VEATE EM Controllers/TEEM Power/TEEM Power/TEEM - HC LS CR ==
  note: MAKE SURE WE DON"T EXTRACT NET POWER DURING THE ACCEL
  note: HP EM
  note: LP EM
  note: HP - CARRIER , LP - SUN, COUPLING - RING
  note: COUPLING EM
  PwrInAccel : Inport
  PwrExAccel : Inport  Port=2
  PwrXDecel : Inport  Port=3
  K_PXeffH : Inport  Port=4
  K_PXeffL : Inport  Port=5
  transientType : Inport  Port=6
  Abs : Abs  SaturateOnIntegerOverflow=off
  Abs1 : Abs  SaturateOnIntegerOverflow=off
  Abs2 : Abs  SaturateOnIntegerOverflow=off
  Divide : Product  Inputs=*/
  Divide{2,5,9,11} (4 alike) : Product  Inputs=**
  Divide4 : Product  Inputs=*/
  Divide6 : Product  Inputs=*/
  Gain : Gain  Gain=-1
  Gain2 : Gain  Gain=-1
  Gain3 : Gain  Gain=-1
  MinMax : MinMax
  MinMax2 : MinMax
  Mux1 : Mux  Inputs=2
  Mux3 : Mux  Inputs=2
  PwrMax_TEEM : Constant  Value=MWS.PowerSystem.PwrMaxCoup_TEEMa
  PwrMax_TEEM1 : Constant  Value=MWS.PowerSystem.PwrMaxH_TEEM  VectorParams1D=off
  PwrMax_TEEM2 : Constant  Value=MWS.PowerSystem.PwrMaxCoup_TEEMd
  Rate Limiter : RateLimiter  RisingSlewLimit=inf  FallingSlewLimit=-MWS.PowerSystem.PwrMaxCoup_TEEMa/0.8  SampleTimeMode=inherited
  Relational Operator : RelationalOperator  Operator=>  OutDataTypeStr=boolean  RndMeth=Simplest  InputSameDT=off
  Sign : Signum
  Sign2 : Signum
  Sum1 : Sum  Inputs=|-+
  Sum2 : Sum  Inputs=|-+
  Sum3 : Sum  Inputs=|+-
  Sum4 : Sum  Inputs=|+-
  Switch{,1..4} (5 alike) : Switch  Criteria=u2 > Threshold  SaturateOnIntegerOverflow=off  InputSameDT=off
  Terminator : Terminator
  Terminator1 : Terminator
  Zero : Constant  Value=0
  Zero1 : Constant
  Zero2 : Constant
  zero : Constant  Value=0
  PemS_TEEM : Outport
  PemR_TEEM : Outport  Port=2
  PemC_TEEM : Outport  Port=3
  PemP_TEEM : Outport  Port=4
  wires:
  [PwrXDecel] -> Divide4/1
  Sum4/1 -> Divide4/2
  [K_PXeffH] -> Sum4/2
  Zero2/1 -> Sum4/1
  Divide4/1 -> Gain3/1
  Gain3/1 -> Switch/3
  [transientType] -> Switch4/2
  Switch4/1 -> PemR_TEEM/1, [PemCoup_Base]  "Power of Coupling EM"
  Gain2/1 -> Switch3/1
  Abs1/1 -> Relational Operator/1
  Divide6/1 -> Gain2/1
  [PwrInAccel] -> Divide6/1
  Sum3/1 -> Divide6/2
  [K_PXeffH] -> Sum3/2
  Zero1/1 -> Sum3/1
  Switch3/1 -> Switch4/1
  Relational Operator/1 -> Switch3/2
  Sum2/1 -> Relational Operator/2  "PH"
  Divide5/1 -> Sum2/1  "PwrXL2H"
  [PwrInAccel] -> Sum2/2
  Rate Limiter/1 -> Abs1/1, Divide5/1, Switch3/3  "PCoup"
  [K_PXeffH] -> Divide5/2
  [PwrInAccel] -> Divide/1
  [PemCoup_Base] -> Divide9/1, Gain/1
  PwrExAccel/1 -> Terminator/1
  Divide/1 -> Switch/1
  K_PXeffL/1 -> Terminator1/1
  [transientType] -> Switch2/2, Switch/2
  PwrMax_TEEM2/1 -> Switch2/3
  PwrMax_TEEM/1 -> Switch2/1
  Switch2/1 -> Mux1/2
  Gain/1 -> Switch1/3
  [transientType] -> Switch1/2
  Sum1/1 -> Switch1/1
  transientType/1 -> [transientType]
  [K_PXeffH] -> Divide9/2
  [K_PXeffH] -> Divide/2
  K_PXeffH/1 -> [K_PXeffH]
  PwrXDecel/1 -> [PwrXDecel]
  PwrInAccel/1 -> [PwrInAccel]
  Divide2/1 -> Switch4/3, Rate Limiter/1
  Zero/1 -> PemP_TEEM/1
  [PwrInAccel] -> Sum1/2
  Divide9/1 -> Sum1/1
  Sign2/1 -> Divide11/1
  Sign/1 -> Divide2/1
  MinMax2/1 -> Divide11/2
  Divide11/1 -> PemC_TEEM/1
  Mux1/1 -> Abs/1
  Abs2/1 -> MinMax2/1
  Switch1/1 -> Sign2/1, Mux3/1
  MinMax/1 -> Divide2/2
  Switch/1 -> Mux1/1, Sign/1  "Power of Coupling EM"
  Mux3/1 -> Abs2/1
  zero/1 -> PemS_TEEM/1
  PwrMax_TEEM1/1 -> Mux3/2
  Abs/1 -> MinMax/1

== system AGTF30SysDyn_PExPIn/Control System/Electric Machine Controllers/EM Controllers/PGB EM Control/VEATE EM Controllers/TEEM Power/TEEM Power/TEEM - HR LC CS ==
  note: HP EM
  note: LP EM
  note: HP - RING, LP - CARRIER , COUPLING - SUN
  note: COUPLING EM
  PwrInAccel : Inport
  PwrExAccel : Inport  Port=2
  PwrXDecel : Inport  Port=3
  K_PXeffH : Inport  Port=4
  K_PXeffL : Inport  Port=5
  transientType : Inport  Port=6
  Abs : Abs  SaturateOnIntegerOverflow=off
  Abs1 : Abs  SaturateOnIntegerOverflow=off
  Abs2 : Abs  SaturateOnIntegerOverflow=off
  Divide : Product  Inputs=*/
  Divide{2,5,9,11} (4 alike) : Product  Inputs=**
  Divide4 : Product  Inputs=*/
  Divide6 : Product  Inputs=*/
  Gain : Gain  Gain=-1
  Gain2 : Gain  Gain=-1
  Gain3 : Gain  Gain=-1
  MinMax : MinMax
  MinMax2 : MinMax
  Mux1 : Mux  Inputs=2
  Mux3 : Mux  Inputs=2
  PwrMax_TEEM : Constant  Value=MWS.PowerSystem.PwrMaxCoup_TEEMa
  PwrMax_TEEM1 : Constant  Value=MWS.PowerSystem.PwrMaxH_TEEM  VectorParams1D=off
  PwrMax_TEEM2 : Constant  Value=MWS.PowerSystem.PwrMaxCoup_TEEMd
  Rate Limiter : RateLimiter  RisingSlewLimit=inf  FallingSlewLimit=-MWS.PowerSystem.PwrMaxCoup_TEEMa/0.8  SampleTimeMode=inherited
  Relational Operator : RelationalOperator  Operator=>  OutDataTypeStr=boolean  RndMeth=Simplest  InputSameDT=off
  Sign : Signum
  Sign2 : Signum
  Sum1 : Sum  Inputs=|-+
  Sum2 : Sum  Inputs=|-+
  Sum3 : Sum  Inputs=|+-
  Sum4 : Sum  Inputs=|+-
  Switch{,1..4} (5 alike) : Switch  Criteria=u2 > Threshold  SaturateOnIntegerOverflow=off  InputSameDT=off
  Terminator : Terminator
  Terminator1 : Terminator
  Zero : Constant  Value=0
  Zero1 : Constant
  Zero2 : Constant
  zero : Constant  Value=0
  PemS_TEEM : Outport
  PemR_TEEM : Outport  Port=2
  PemC_TEEM : Outport  Port=3
  PemP_TEEM : Outport  Port=4
  wires:
  [PwrXDecel] -> Divide4/1
  Sum4/1 -> Divide4/2
  [K_PXeffH] -> Sum4/2
  Zero2/1 -> Sum4/1
  Divide4/1 -> Gain3/1
  Gain3/1 -> Switch/3
  [transientType] -> Switch4/2
  Switch4/1 -> PemS_TEEM/1, [PemCoup_Base]  "Power of Coupling EM"
  Gain2/1 -> Switch3/1
  Abs1/1 -> Relational Operator/1
  Divide6/1 -> Gain2/1
  [PwrInAccel] -> Divide6/1
  Sum3/1 -> Divide6/2
  [K_PXeffH] -> Sum3/2
  Zero1/1 -> Sum3/1
  Switch3/1 -> Switch4/1
  Relational Operator/1 -> Switch3/2
  Sum2/1 -> Relational Operator/2  "PH"
  Divide5/1 -> Sum2/1  "PwrXL2H"
  [PwrInAccel] -> Sum2/2
  Rate Limiter/1 -> Abs1/1, Divide5/1, Switch3/3  "PCoup"
  [K_PXeffH] -> Divide5/2
  [PwrInAccel] -> Divide/1
  [PemCoup_Base] -> Divide9/1, Gain/1
  PwrExAccel/1 -> Terminator/1
  Divide/1 -> Switch/1
  K_PXeffL/1 -> Terminator1/1
  [transientType] -> Switch2/2, Switch/2
  PwrMax_TEEM2/1 -> Switch2/3
  PwrMax_TEEM/1 -> Switch2/1
  Switch2/1 -> Mux1/2
  Gain/1 -> Switch1/3
  [transientType] -> Switch1/2
  Sum1/1 -> Switch1/1
  transientType/1 -> [transientType]
  [K_PXeffH] -> Divide9/2
  [K_PXeffH] -> Divide/2
  K_PXeffH/1 -> [K_PXeffH]
  PwrXDecel/1 -> [PwrXDecel]
  PwrInAccel/1 -> [PwrInAccel]
  Divide2/1 -> Switch4/3, Rate Limiter/1
  Zero/1 -> PemP_TEEM/1
  [PwrInAccel] -> Sum1/2
  Divide9/1 -> Sum1/1
  Sign2/1 -> Divide11/1
  Sign/1 -> Divide2/1
  MinMax2/1 -> Divide11/2
  Divide11/1 -> PemR_TEEM/1
  Mux1/1 -> Abs/1
  Abs2/1 -> MinMax2/1
  Switch1/1 -> Sign2/1, Mux3/1
  MinMax/1 -> Divide2/2
  Switch/1 -> Mux1/1, Sign/1  "Power of Coupling EM"
  Mux3/1 -> Abs2/1
  zero/1 -> PemC_TEEM/1
  PwrMax_TEEM1/1 -> Mux3/2
  Abs/1 -> MinMax/1

== system AGTF30SysDyn_PExPIn/Control System/Electric Machine Controllers/EM Controllers/PGB EM Control/VEATE EM Controllers/TEEM Power/TEEM Power/TEEM - HR LS CC ==
  note: HP EM
  note: LP EM
  note: HP - RING , LP - SUN, COUPLING - CARRIER
  note: COUPLING EM
  PwrInAccel : Inport
  PwrExAccel : Inport  Port=2
  PwrXDecel : Inport  Port=3
  K_PXeffH : Inport  Port=4
  K_PXeffL : Inport  Port=5
  transientType : Inport  Port=6
  Abs : Abs  SaturateOnIntegerOverflow=off
  Abs1 : Abs  SaturateOnIntegerOverflow=off
  Abs2 : Abs  SaturateOnIntegerOverflow=off
  Divide : Product  Inputs=*/
  Divide{2,5,9,11} (4 alike) : Product  Inputs=**
  Divide4 : Product  Inputs=*/
  Divide6 : Product  Inputs=*/
  Gain : Gain  Gain=-1
  Gain2 : Gain  Gain=-1
  Gain3 : Gain  Gain=-1
  MinMax : MinMax
  MinMax2 : MinMax
  Mux1 : Mux  Inputs=2
  Mux3 : Mux  Inputs=2
  PwrMax_TEEM : Constant  Value=MWS.PowerSystem.PwrMaxCoup_TEEMa
  PwrMax_TEEM1 : Constant  Value=MWS.PowerSystem.PwrMaxH_TEEM  VectorParams1D=off
  PwrMax_TEEM2 : Constant  Value=MWS.PowerSystem.PwrMaxCoup_TEEMd
  Rate Limiter : RateLimiter  RisingSlewLimit=inf  FallingSlewLimit=-MWS.PowerSystem.PwrMaxCoup_TEEMa/0.8  SampleTimeMode=inherited
  Relational Operator : RelationalOperator  Operator=>  OutDataTypeStr=boolean  RndMeth=Simplest  InputSameDT=off
  Sign : Signum
  Sign2 : Signum
  Sum1 : Sum  Inputs=|-+
  Sum2 : Sum  Inputs=|-+
  Sum3 : Sum  Inputs=|+-
  Sum4 : Sum  Inputs=|+-
  Switch{,1..4} (5 alike) : Switch  Criteria=u2 > Threshold  SaturateOnIntegerOverflow=off  InputSameDT=off
  Terminator : Terminator
  Terminator1 : Terminator
  Zero : Constant  Value=0
  Zero1 : Constant
  Zero2 : Constant
  zero : Constant  Value=0
  PemS_TEEM : Outport
  PemR_TEEM : Outport  Port=2
  PemC_TEEM : Outport  Port=3
  PemP_TEEM : Outport  Port=4
  wires:
  [PwrXDecel] -> Divide4/1
  Sum4/1 -> Divide4/2
  [K_PXeffH] -> Sum4/2
  Zero2/1 -> Sum4/1
  Divide4/1 -> Gain3/1
  Gain3/1 -> Switch/3
  [transientType] -> Switch4/2
  Switch4/1 -> [PemCoup_Base], PemC_TEEM/1  "Power of Coupling EM"
  Gain2/1 -> Switch3/1
  Abs1/1 -> Relational Operator/1
  Divide6/1 -> Gain2/1
  [PwrInAccel] -> Divide6/1
  Sum3/1 -> Divide6/2
  [K_PXeffH] -> Sum3/2
  Zero1/1 -> Sum3/1
  Switch3/1 -> Switch4/1
  Relational Operator/1 -> Switch3/2
  Sum2/1 -> Relational Operator/2  "PH"
  Divide5/1 -> Sum2/1  "PwrXL2H"
  [PwrInAccel] -> Sum2/2
  Rate Limiter/1 -> Abs1/1, Divide5/1, Switch3/3  "PCoup"
  [K_PXeffH] -> Divide5/2
  [PwrInAccel] -> Divide/1
  [PemCoup_Base] -> Divide9/1, Gain/1
  PwrExAccel/1 -> Terminator/1
  Divide/1 -> Switch/1
  K_PXeffL/1 -> Terminator1/1
  [transientType] -> Switch2/2, Switch/2
  PwrMax_TEEM2/1 -> Switch2/3
  PwrMax_TEEM/1 -> Switch2/1
  Switch2/1 -> Mux1/2
  Gain/1 -> Switch1/3
  [transientType] -> Switch1/2
  Sum1/1 -> Switch1/1
  transientType/1 -> [transientType]
  [K_PXeffH] -> Divide9/2
  [K_PXeffH] -> Divide/2
  K_PXeffH/1 -> [K_PXeffH]
  PwrXDecel/1 -> [PwrXDecel]
  PwrInAccel/1 -> [PwrInAccel]
  Divide2/1 -> Switch4/3, Rate Limiter/1
  Zero/1 -> PemP_TEEM/1
  [PwrInAccel] -> Sum1/2
  Divide9/1 -> Sum1/1
  Sign2/1 -> Divide11/1
  Sign/1 -> Divide2/1
  MinMax2/1 -> Divide11/2
  Divide11/1 -> PemR_TEEM/1
  Mux1/1 -> Abs/1
  Abs2/1 -> MinMax2/1
  Switch1/1 -> Sign2/1, Mux3/1
  MinMax/1 -> Divide2/2
  Switch/1 -> Mux1/1, Sign/1  "Power of Coupling EM"
  Mux3/1 -> Abs2/1
  zero/1 -> PemS_TEEM/1
  PwrMax_TEEM1/1 -> Mux3/2
  Abs/1 -> MinMax/1

== system AGTF30SysDyn_PExPIn/Control System/Electric Machine Controllers/EM Controllers/PGB EM Control/VEATE EM Controllers/TEEM Power/TEEM Power/TEEM - HS LC CR ==
  note: COUPLING EM
  note: HP - SUN, LP - CARRIER, COUPLING - RING
  note: LP EM
  note: HP EM
  PwrInAccel : Inport
  PwrExAccel : Inport  Port=2
  PwrXDecel : Inport  Port=3
  K_PXeffH : Inport  Port=4
  K_PXeffL : Inport  Port=5
  transientType : Inport  Port=6
  Abs : Abs  SaturateOnIntegerOverflow=off
  Abs1 : Abs  SaturateOnIntegerOverflow=off
  Abs2 : Abs  SaturateOnIntegerOverflow=off
  Divide : Product  Inputs=*/
  Divide{2,5,9,11} (4 alike) : Product  Inputs=**
  Divide4 : Product  Inputs=*/
  Divide6 : Product  Inputs=*/
  Gain : Gain  Gain=-1
  Gain2 : Gain  Gain=-1
  Gain3 : Gain  Gain=-1
  MinMax : MinMax
  MinMax2 : MinMax
  Mux1 : Mux  Inputs=2
  Mux3 : Mux  Inputs=2
  PwrMax_TEEM : Constant  Value=MWS.PowerSystem.PwrMaxCoup_TEEMa
  PwrMax_TEEM1 : Constant  Value=MWS.PowerSystem.PwrMaxH_TEEM  VectorParams1D=off
  PwrMax_TEEM2 : Constant  Value=MWS.PowerSystem.PwrMaxCoup_TEEMd
  Rate Limiter : RateLimiter  RisingSlewLimit=inf  FallingSlewLimit=-MWS.PowerSystem.PwrMaxCoup_TEEMa/0.8  SampleTimeMode=inherited
  Relational Operator : RelationalOperator  Operator=>  OutDataTypeStr=boolean  RndMeth=Simplest  InputSameDT=off
  Sign : Signum
  Sign2 : Signum
  Sum1 : Sum  Inputs=|-+
  Sum2 : Sum  Inputs=|-+
  Sum3 : Sum  Inputs=|+-
  Sum4 : Sum  Inputs=|+-
  Switch{,1..4} (5 alike) : Switch  Criteria=u2 > Threshold  SaturateOnIntegerOverflow=off  InputSameDT=off
  Terminator : Terminator
  Terminator1 : Terminator
  Zero : Constant  Value=0
  Zero1 : Constant
  Zero2 : Constant
  zero : Constant  Value=0
  PemS_TEEM : Outport
  PemR_TEEM : Outport  Port=2
  PemC_TEEM : Outport  Port=3
  PemP_TEEM : Outport  Port=4
  wires:
  Abs/1 -> MinMax/1
  PwrMax_TEEM1/1 -> Mux3/2
  zero/1 -> PemC_TEEM/1
  Mux3/1 -> Abs2/1
  Switch/1 -> Sign/1, Mux1/1  "Power of Coupling EM"
  MinMax/1 -> Divide2/2
  Switch1/1 -> Mux3/1, Sign2/1
  Abs2/1 -> MinMax2/1
  Mux1/1 -> Abs/1
  Divide11/1 -> PemS_TEEM/1
  MinMax2/1 -> Divide11/2
  Sign/1 -> Divide2/1
  Sign2/1 -> Divide11/1
  Divide9/1 -> Sum1/1
  [PwrInAccel] -> Sum1/2
  Zero/1 -> PemP_TEEM/1
  Divide2/1 -> Rate Limiter/1, Switch4/3
  PwrInAccel/1 -> [PwrInAccel]
  PwrXDecel/1 -> [PwrXDecel]
  K_PXeffH/1 -> [K_PXeffH]
  [K_PXeffH] -> Divide/2
  [K_PXeffH] -> Divide9/2
  transientType/1 -> [transientType]
  Sum1/1 -> Switch1/1
  [transientType] -> Switch1/2
  Gain/1 -> Switch1/3
  Switch2/1 -> Mux1/2
  PwrMax_TEEM/1 -> Switch2/1
  PwrMax_TEEM2/1 -> Switch2/3
  [transientType] -> Switch/2, Switch2/2
  K_PXeffL/1 -> Terminator1/1
  Divide/1 -> Switch/1
  PwrExAccel/1 -> Terminator/1
  [PemCoup_Base] -> Gain/1, Divide9/1
  [PwrInAccel] -> Divide/1
  [K_PXeffH] -> Divide5/2
  Rate Limiter/1 -> Switch3/3, Divide5/1, Abs1/1  "PCoup"
  [PwrInAccel] -> Sum2/2
  Divide5/1 -> Sum2/1  "PwrXL2H"
  Sum2/1 -> Relational Operator/2  "PH"
  Relational Operator/1 -> Switch3/2
  Switch3/1 -> Switch4/1
  Zero1/1 -> Sum3/1
  [K_PXeffH] -> Sum3/2
  Sum3/1 -> Divide6/2
  [PwrInAccel] -> Divide6/1
  Divide6/1 -> Gain2/1
  Abs1/1 -> Relational Operator/1
  Gain2/1 -> Switch3/1
  Switch4/1 -> [PemCoup_Base], PemR_TEEM/1  "Power of Coupling EM"
  [transientType] -> Switch4/2
  Gain3/1 -> Switch/3
  Divide4/1 -> Gain3/1
  Zero2/1 -> Sum4/1
  [K_PXeffH] -> Sum4/2
  Sum4/1 -> Divide4/2
  [PwrXDecel] -> Divide4/1

== system AGTF30SysDyn_PExPIn/Control System/Electric Machine Controllers/EM Controllers/PGB EM Control/VEATE EM Controllers/TEEM Power/TEEM Power/TEEM - HS LR CC ==
  note: HP EM
  note: LP EM
  note: HP - SUN, LP - RING, COUPLING - CARRIER
  note: COUPLING EM
  PwrInAccel : Inport
  PwrExAccel : Inport  Port=2
  PwrXDecel : Inport  Port=3
  K_PXeffH : Inport  Port=4
  K_PXeffL : Inport  Port=5
  transientType : Inport  Port=6
  Abs : Abs  SaturateOnIntegerOverflow=off
  Abs1 : Abs  SaturateOnIntegerOverflow=off
  Abs2 : Abs  SaturateOnIntegerOverflow=off
  Divide : Product  Inputs=*/
  Divide{2,5,9,11} (4 alike) : Product  Inputs=**
  Divide4 : Product  Inputs=*/
  Divide6 : Product  Inputs=*/
  Gain : Gain  Gain=-1
  Gain2 : Gain  Gain=-1
  Gain3 : Gain  Gain=-1
  MinMax : MinMax
  MinMax2 : MinMax
  Mux1 : Mux  Inputs=2
  Mux3 : Mux  Inputs=2
  PwrMax_TEEM : Constant  Value=MWS.PowerSystem.PwrMaxCoup_TEEMa
  PwrMax_TEEM1 : Constant  Value=MWS.PowerSystem.PwrMaxH_TEEM  VectorParams1D=off
  PwrMax_TEEM2 : Constant  Value=MWS.PowerSystem.PwrMaxCoup_TEEMd
  Rate Limiter : RateLimiter  RisingSlewLimit=inf  FallingSlewLimit=-MWS.PowerSystem.PwrMaxCoup_TEEMa/0.8  SampleTimeMode=inherited
  Relational Operator : RelationalOperator  Operator=>  OutDataTypeStr=boolean  RndMeth=Simplest  InputSameDT=off
  Sign : Signum
  Sign2 : Signum
  Sum1 : Sum  Inputs=|-+
  Sum2 : Sum  Inputs=|-+
  Sum3 : Sum  Inputs=|+-
  Sum4 : Sum  Inputs=|+-
  Switch{,1..4} (5 alike) : Switch  Criteria=u2 > Threshold  SaturateOnIntegerOverflow=off  InputSameDT=off
  Terminator : Terminator
  Terminator1 : Terminator
  Zero : Constant  Value=0
  Zero1 : Constant
  Zero2 : Constant
  zero : Constant  Value=0
  PemS_TEEM : Outport
  PemR_TEEM : Outport  Port=2
  PemC_TEEM : Outport  Port=3
  PemP_TEEM : Outport  Port=4
  wires:
  [PwrXDecel] -> Divide4/1
  Sum4/1 -> Divide4/2
  [K_PXeffH] -> Sum4/2
  Zero2/1 -> Sum4/1
  Divide4/1 -> Gain3/1
  Gain3/1 -> Switch/3
  [transientType] -> Switch4/2
  Switch4/1 -> PemC_TEEM/1, [PemCoup_Base]  "Power of Coupling EM"
  Gain2/1 -> Switch3/1
  Abs1/1 -> Relational Operator/1
  Divide6/1 -> Gain2/1
  [PwrInAccel] -> Divide6/1
  Sum3/1 -> Divide6/2
  [K_PXeffH] -> Sum3/2
  Zero1/1 -> Sum3/1
  Switch3/1 -> Switch4/1
  Relational Operator/1 -> Switch3/2
  Sum2/1 -> Relational Operator/2  "PH"
  Divide5/1 -> Sum2/1  "PwrXL2H"
  [PwrInAccel] -> Sum2/2
  Rate Limiter/1 -> Abs1/1, Divide5/1, Switch3/3  "PCoup"
  [K_PXeffH] -> Divide5/2
  [PwrInAccel] -> Divide/1
  [PemCoup_Base] -> Divide9/1, Gain/1
  PwrExAccel/1 -> Terminator/1
  Divide/1 -> Switch/1
  K_PXeffL/1 -> Terminator1/1
  [transientType] -> Switch2/2, Switch/2
  PwrMax_TEEM2/1 -> Switch2/3
  PwrMax_TEEM/1 -> Switch2/1
  Switch2/1 -> Mux1/2
  Gain/1 -> Switch1/3
  [transientType] -> Switch1/2
  Sum1/1 -> Switch1/1
  transientType/1 -> [transientType]
  [K_PXeffH] -> Divide9/2
  [K_PXeffH] -> Divide/2
  K_PXeffH/1 -> [K_PXeffH]
  PwrXDecel/1 -> [PwrXDecel]
  PwrInAccel/1 -> [PwrInAccel]
  Divide2/1 -> Switch4/3, Rate Limiter/1
  Zero/1 -> PemP_TEEM/1
  [PwrInAccel] -> Sum1/2
  Divide9/1 -> Sum1/1
  Sign2/1 -> Divide11/1
  Sign/1 -> Divide2/1
  MinMax2/1 -> Divide11/2
  Divide11/1 -> PemS_TEEM/1
  Mux1/1 -> Abs/1
  Abs2/1 -> MinMax2/1
  Switch1/1 -> Sign2/1, Mux3/1
  MinMax/1 -> Divide2/2
  Switch/1 -> Mux1/1, Sign/1  "Power of Coupling EM"
  Mux3/1 -> Abs2/1
  zero/1 -> PemR_TEEM/1
  PwrMax_TEEM1/1 -> Mux3/2
  Abs/1 -> MinMax/1

== matlab function AGTF30SysDyn_PExPIn/Actuators/LPS Electric Machine/Rate Limit Enforcement ==
  data: M_preRL input; M_act output; M_old input; Mdot_low input; Mdot_hi input; dt input
function M_act  = fcn(M_preRL,M_old,Mdot_low,Mdot_hi,dt)

M_act = M_preRL;
if (M_preRL < 0 && M_old > 0) || (M_preRL > 0 && M_old < 0)
    M_act = 0;
elseif M_preRL >= 0
    if (M_preRL-M_old)/dt > Mdot_hi
        M_act = M_old + Mdot_hi*dt;
    else
        M_act = M_preRL;
    end
elseif M_preRL < 0
    if (M_preRL-M_old)/dt < Mdot_low
        M_act = M_old + Mdot_low*dt;
    else
        M_act = M_preRL;
    end
end

== matlab function AGTF30SysDyn_PExPIn/Actuators/HPS Electric Machine/Rate Limit Enforcement ==
  data: M_preRL input; M_act output; M_old input; Mdot_low input; Mdot_hi input; dt input
function M_act  = fcn(M_preRL,M_old,Mdot_low,Mdot_hi,dt)

M_act = M_preRL;
if (M_preRL < 0 && M_old > 0) || (M_preRL > 0 && M_old < 0)
    M_act = 0;
elseif M_preRL >= 0
    if (M_preRL-M_old)/dt > Mdot_hi
        M_act = M_old + Mdot_hi*dt;
    else
        M_act = M_preRL;
    end
elseif M_preRL < 0
    if (M_preRL-M_old)/dt < Mdot_low
        M_act = M_old + Mdot_low*dt;
    else
        M_act = M_preRL;
    end
end

== matlab function AGTF30SysDyn_PExPIn/Actuators/Sun Gear Electric Machine/Rate Limit Enforcement ==
  data: M_preRL input; M_act output; M_old input; Mdot_low input; Mdot_hi input; dt input
function M_act  = fcn(M_preRL,M_old,Mdot_low,Mdot_hi,dt)

M_act = M_preRL;
if (M_preRL < 0 && M_old > 0) || (M_preRL > 0 && M_old < 0)
    M_act = 0;
elseif M_preRL >= 0
    if (M_preRL-M_old)/dt > Mdot_hi
        M_act = M_old + Mdot_hi*dt;
    else
        M_act = M_preRL;
    end
elseif M_preRL < 0
    if (M_preRL-M_old)/dt < Mdot_low
        M_act = M_old + Mdot_low*dt;
    else
        M_act = M_preRL;
    end
end
